simulink model "Clase_parcial_2_control_2_seguidor"  (R2016a)
settings: Solver=VariableStepAuto  StartTime=0.0  StopTime=10.0  RelTol=1e-3
values from neighbouring files (symbols this model uses):
  A = [0,1;19,1]    [Control_sist_no_lineal_punto_operacion.m]    (also in Datos_Regulador_Segundo_Orden.mat = [-1  0; 0  2]; Metodo_ganancias.m = [0,1;3*x.^2+10*x+6,1]; Metodo_modos_deslizantes.m = [0 1;-12 -7]; Observador_Estados.m = [-1,0;0,2])
  B = [1;2]    [Control_sist_no_lineal_punto_operacion.m]    (also in Datos_Regulador_Segundo_Orden.mat = [1 1]; Metodo_ganancias.m; Metodo_modos_deslizantes.m = [0;1]; Observador_Estados.m = [1;1])
  C = [1,0]    [Control_sist_no_lineal_punto_operacion.m]    (also in Datos_Regulador_Segundo_Orden.mat = [1 1]; Metodo_ganancias.m; Metodo_modos_deslizantes.m = [1 0]; Observador_Estados.m = [1,1])
  ki = k(1:1,3:3)    [Control_sist_no_lineal_punto_operacion.m]    (also in Observador_Estados_codigo_matlab.m = k(:,3:3))
  kp = k(1:1,1:2)    [Control_sist_no_lineal_punto_operacion.m]    (also in Observador_Estados_codigo_matlab.m = k(:,1:2))
settings Model: Creator=Daniel  LastModifiedBy=Daniel

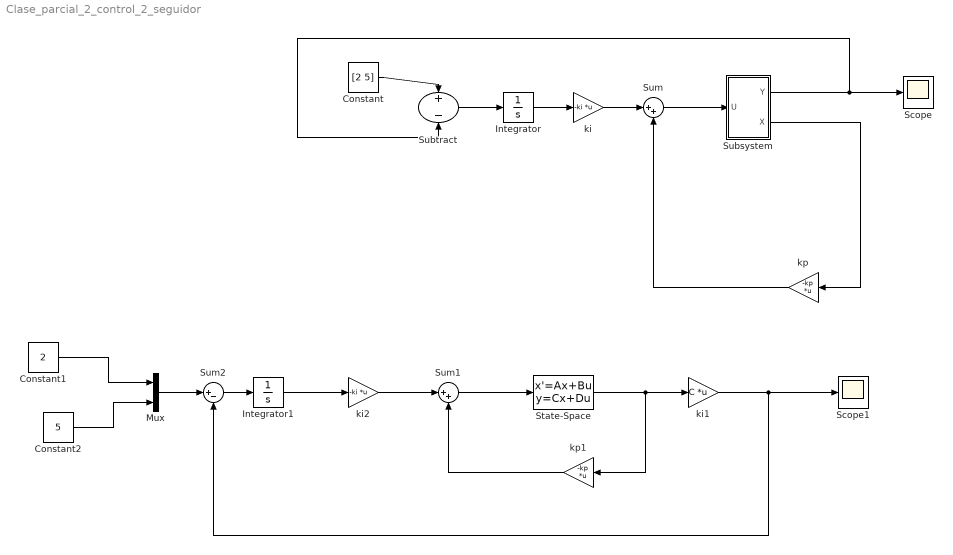
== system Clase_parcial_2_control_2_seguidor ==
  Constant : Constant  Value=[2 5]
  Constant1 : Constant  Value=2
  Constant2 : Constant  Value=5
  Integrator : Integrator
  Integrator1 : Integrator
  Mux : Mux  Inputs=2
  Scope : Scope
  Scope1 : Scope
  State-Space : StateSpace  A=A  B=B  C=eye(2)  D=zeros(2,2)  X0=0
  Subsystem : Subsystem
  Subtract : Sum  Inputs=+-
  Sum : Sum  Inputs=|++
  Sum1 : Sum  Inputs=|++
  Sum2 : Sum  Inputs=|+-
  ki : Gain  Gain=-ki  Multiplication=Matrix(K*u) (u vector)
  ki1 : Gain  Gain=C  Multiplication=Matrix(K*u) (u vector)
  ki2 : Gain  Gain=-ki  Multiplication=Matrix(K*u) (u vector)
  kp : Gain  Gain=-kp  Multiplication=Matrix(K*u) (u vector)
  kp1 : Gain  Gain=-kp  Multiplication=Matrix(K*u) (u vector)
  wires:
  Subsystem/1(Y) -> Subtract/2, Scope/1
  Subsystem/2(X) -> kp/1
  Constant/1 -> Subtract/1
  Subtract/1 -> Integrator/1
  Integrator/1 -> ki/1
  ki/1 -> Sum/1
  kp/1 -> Sum/2
  Sum/1 -> Subsystem/1(U)
  Sum1/1 -> State-Space/1
  kp1/1 -> Sum1/2
  ki2/1 -> Sum1/1
  Integrator1/1 -> ki2/1
  Sum2/1 -> Integrator1/1
  Mux/1 -> Sum2/1
  State-Space/1 -> ki1/1, kp1/1
  Constant2/1 -> Mux/2
  Constant1/1 -> Mux/1
  ki1/1 -> Sum2/2, Scope1/1

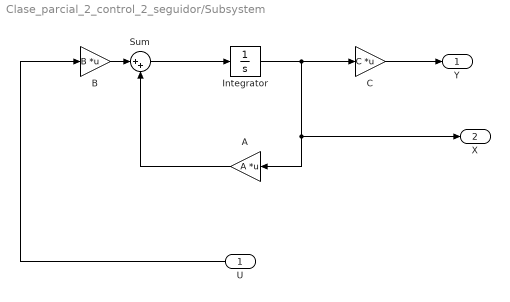
== system Clase_parcial_2_control_2_seguidor/Subsystem ==
  U : Inport
  A : Gain  Gain=A  Multiplication=Matrix(K*u) (u vector)
  B : Gain  Gain=B  Multiplication=Matrix(K*u) (u vector)
  C : Gain  Gain=C  Multiplication=Matrix(K*u) (u vector)
  Integrator : Integrator
  Sum : Sum  Inputs=|++
  Y : Outport
  X : Outport  Port=2
  wires:
  Sum/1 -> Integrator/1
  A/1 -> Sum/2
  U/1 -> B/1
  B/1 -> Sum/1
  C/1 -> Y/1
  Integrator/1 -> X/1, A/1, C/1
